simulink model "valve_test"  (R2021a)
settings: Solver=VariableStepAuto  StartTime=0.0  StopTime=10.0  RelTol=1e-3
undefined symbols (not defined in the file or in its folder): lookup_n, lookup_q_l
libraries: simulink x2
settings Model: Creator=artof  LastModifiedBy=artof

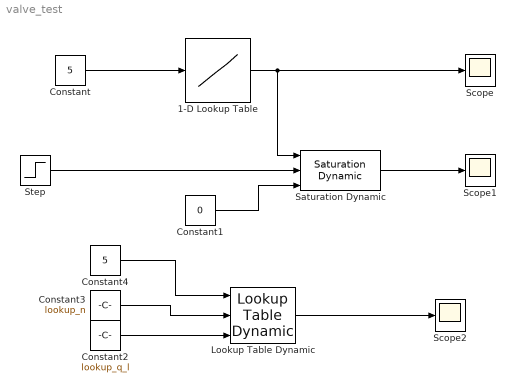
== system valve_test ==
  1-D Lookup Table : Lookup_n-D  NumberOfTableDimensions=1  BreakpointsForDimension1=[1 2 3 4 5 6 7 8 9 10]  Table=[130 80 50 35 20 15 10 7 5 3]  TableDataTypeStr=double  InternalRulePriority=Speed  RndMeth=Simplest  InputSameDT=on
  Constant : Constant  Value=5
  Constant1 : Constant  Value=0
  Constant2 : Constant  Value=lookup_q_l
  Constant3 : Constant  Value=lookup_n
  Constant4 : Constant  Value=5
  Lookup Table Dynamic : simulink/Lookup Tables/Lookup Table Dynamic  LookUpMeth=Interpolation-Use End Values  OutDataType=fixdt('double')  OutScaling=2^-10  OutputDataTypeScalingMode=Specify via dialog  OutDataTypeStr=double  DoSatur=off
  Saturation Dynamic : simulink/Discontinuities/Saturation Dynamic  OutMin=0  OutMax=[]  OutDataTypeStr=Inherit: Same as second input  OutDataType=fixdt(1, 16)  OutScaling=2^-10  DoSatur=off
  Scope : Scope
  Scope1 : Scope
  Scope2 : Scope
  Step : Step  After=100  SampleTime=0
  wires:
  Constant/1 -> 1-D Lookup Table/1
  1-D Lookup Table/1 -> Saturation Dynamic/1, Scope/1
  Step/1 -> Saturation Dynamic/2
  Constant1/1 -> Saturation Dynamic/3
  Saturation Dynamic/1 -> Scope1/1
  Constant2/1 -> Lookup Table Dynamic/3
  Constant3/1 -> Lookup Table Dynamic/2
  Constant4/1 -> Lookup Table Dynamic/1
  Lookup Table Dynamic/1 -> Scope2/1
